simulink model "VFSIMPLEINVERTER"  (R2022b)
settings: Solver=ode1  StartTime=0.0  StopTime=10.0  FixedStep=1e-4  RelTol=1e-3
values from neighbouring files (symbols this model uses):
  f = 6.32*10.^-4    (= 0.000632)    [VFparam.m]
  J = 4.50*10.^-2    (= 0.045)    [VFparam.m]
  Kim = J*((wnm).^2)/Kpm    [VFparam.m]
  Kpm = 2*wnm*J*ceff-f    (= 2.249368)    [VFparam.m]
  Ktm = 1.5692    [VFparam.m]
  Lr = 0.2395    [VFparam.m]
  Ls = 0.256    [VFparam.m]
  Msr = 0.236    [VFparam.m]
  P = 2    [VFparam.m]
  Rr = 1.09    [VFparam.m]
  Rs = 3.36    [VFparam.m]
  VDC = 1000    [VFparam.m]
  vf = 230*sqrt(2)/50    [VFparam.m]
settings Model: Creator=ZinouAb  LastModifiedBy=ZinouAb

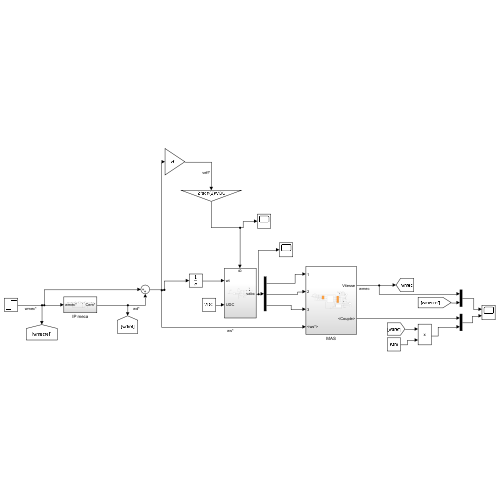
[thumbnail: Simulink's stored preview of the top-level diagram]
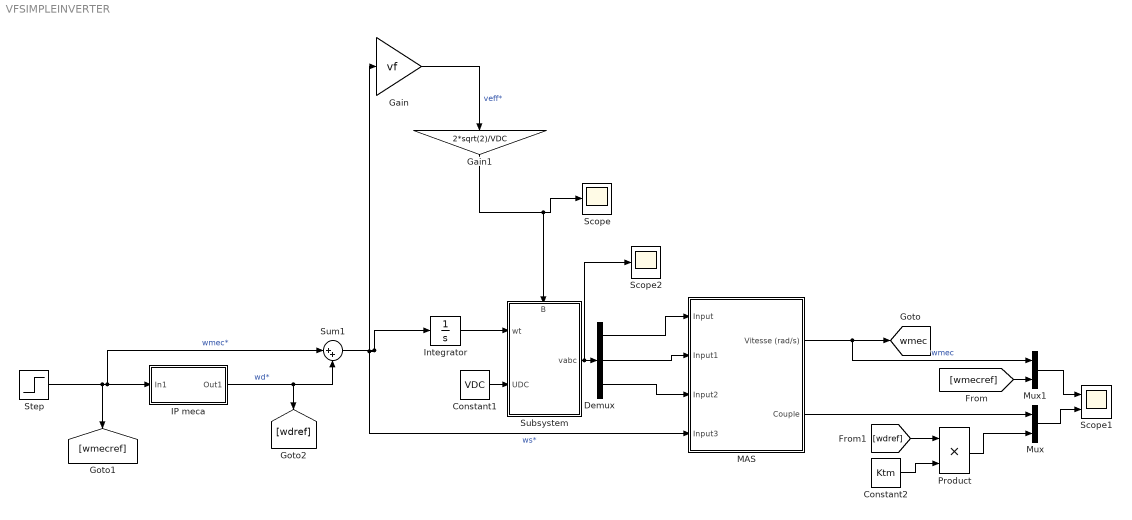
== system VFSIMPLEINVERTER ==
  Constant1 : Constant  Value=VDC
  Constant2 : Constant  Value=Ktm
  Demux : Demux  Outputs=3
  Gain : Gain  Gain=vf
  Gain1 : Gain  Gain=2*sqrt(2)/VDC
  IP meca : Subsystem
  Integrator : Integrator
  MAS : Subsystem
  Mux : Mux  Inputs=2
  Mux1 : Mux  Inputs=2
  Product : Product
  Scope : Scope
  Scope1 : Scope  NumInputPorts=2
  Scope2 : Scope
  Step : Step  Time=4  After=100  SampleTime=0
  Subsystem : Subsystem
      settings: PortSchema="{\"entries\":[{\"content\":{\"sides\":[{\"content\":{\"connectorIds\":[\"In1\",\"In2\"]},\"type\":\"ConnectorPlacement.EquallySpacedRectSide\",\"uuid\":\"b96697a1-7390-4a4c-a090-1d4840f94579\"},{\"content\":{\"connectorIds\":[\"Out1\"],\"side\":\"RIGHT\"},\"type\":\"ConnectorPlacement.EquallySpacedRectSide\",\"uuid\":\"06d1d8c6-d481-421b-9786-6ed8bea33fb5\"},{\"content\":{\"connectorIds\":[\"In3\"],\"side\":\"TOP\"},\"type\":\"ConnectorPlacement.EquallySpacedRectSide\",\"uuid\":\"2e081ee8-1238-4450-99c4-3d0e60d3e391\"}]},\"type\":\"ConnectorPlacement.EquallySpacedConnector\",\"uuid\":\"e9990dc2-fc0c-4c65-980c-f90091d8c920\"}],\"packageUris\":[\"http://schema.mathworks.com/mf0/Connector/R2020b\"],\"version\":\"1.0\"}"
  Sum1 : Sum  Inputs=|++
  tag scope: wmec=global
  wires:
  Step/1 -> IP meca/1(In1), Sum1/1, [wmecref]  "wmec*"
  Gain/1 -> Gain1/1  "veff*"
  Demux/1 -> MAS/1(Input)
  Sum1/1 -> Integrator/1, MAS/4(Input3), Gain/1  "ws*"
  Demux/2 -> MAS/2(Input1)
  MAS/1(Vitesse (rad/s)) -> Mux1/1, [wmec]  "wmec"
  Demux/3 -> MAS/3(Input2)
  IP meca/1(Out1) -> Sum1/2, [wdref]  "wd*"
  Integrator/1 -> Subsystem/1(wt)
  Subsystem/1(vabc) -> Scope2/1, Demux/1
  Constant1/1 -> Subsystem/2(UDC)
  Mux1/1 -> Scope1/1
  Mux/1 -> Scope1/2
  MAS/2(Couple) -> Mux/1
  [wmecref] -> Mux1/2
  [wdref] -> Product/1
  Constant2/1 -> Product/2
  Product/1 -> Mux/2
  Gain1/1 -> Subsystem/3(B), Scope/1

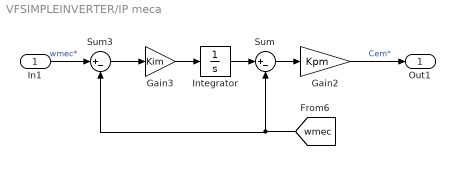
== system VFSIMPLEINVERTER/IP meca ==
  In1 : Inport
  Gain2 : Gain  Gain=Kpm
  Gain3 : Gain  Gain=Kim
  Integrator : Integrator
  Sum : Sum  Inputs=|+-
  Sum3 : Sum  Inputs=|+-
  Out1 : Outport
  wires:
  Integrator/1 -> Sum/1
  [wmec] -> Sum3/2, Sum/2
  Sum/1 -> Gain2/1
  Gain2/1 -> Out1/1  "Cem*"
  Gain3/1 -> Integrator/1
  Sum3/1 -> Gain3/1
  In1/1 -> Sum3/1  "wmec*"

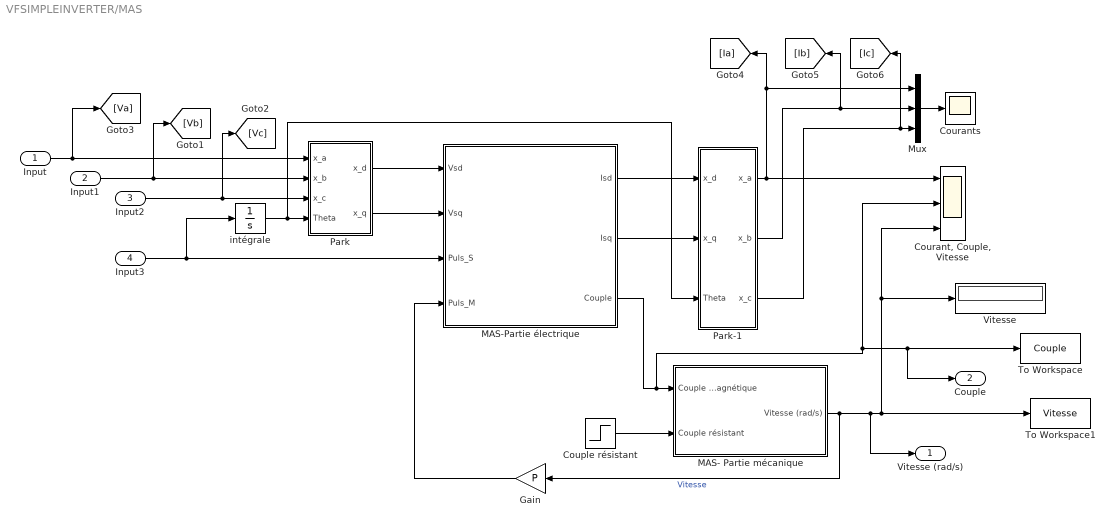
== system VFSIMPLEINVERTER/MAS ==
  Input : Inport
  Input1 : Inport  Port=2
  Input2 : Inport  Port=3
  Input3 : Inport  Port=4
  Couple résistant : Step  Time=6  After=2  SampleTime=0
  "Courant, Couple, Vitesse" : Scope  NumInputPorts=3
  Courants : Scope
  Gain : Gain  Gain=P
  MAS- Partie mécanique : Subsystem
  MAS-Partie électrique : Subsystem
  Mux : Mux  Inputs=3
  Park : Subsystem
  Park-1 : Subsystem
  To Workspace : ToWorkspace  VariableName=Couple  SampleTime=-1
      settings: Save2DSignal=2-D array (concatenate along first dimension)
  To Workspace1 : ToWorkspace  VariableName=Vitesse  SampleTime=-1
      settings: Save2DSignal=2-D array (concatenate along first dimension)
  Vitesse : Display
  intégrale : Integrator
  Vitesse (rad/s) : Outport
  Couple : Outport  Port=2
  wires:
  Park-1/2(x_b) -> [Ib], Mux/2
  Park/2(x_q) -> MAS-Partie électrique/2(Vsq)
  Input2/1 -> [Vc], Park/3(x_c)
  Mux/1 -> Courants/1
  Park-1/1(x_a) -> [Ia], Mux/1, "Courant, Couple, Vitesse"/1
  MAS- Partie mécanique/1(Vitesse (rad/s)) -> Gain/1, Vitesse (rad/s)/1, Vitesse/1, "Courant, Couple, Vitesse"/3, To Workspace1/1  "Vitesse"
  Input/1 -> [Va], Park/1(x_a)
  intégrale/1 -> Park-1/3(Theta), Park/4(Theta)
  MAS-Partie électrique/3(Couple) -> "Courant, Couple, Vitesse"/2, Couple/1, To Workspace/1, MAS- Partie mécanique/1(Couple Electromagnétique)
  Couple résistant/1 -> MAS- Partie mécanique/2(Couple résistant)
  Input1/1 -> [Vb], Park/2(x_b)
  Gain/1 -> MAS-Partie électrique/4(Puls_M)
  Park-1/3(x_c) -> [Ic], Mux/3
  Park/1(x_d) -> MAS-Partie électrique/1(Vsd)
  Input3/1 -> intégrale/1, MAS-Partie électrique/3(Puls_S)
  MAS-Partie électrique/1(Isd) -> Park-1/1(x_d)
  MAS-Partie électrique/2(Isq) -> Park-1/2(x_q)

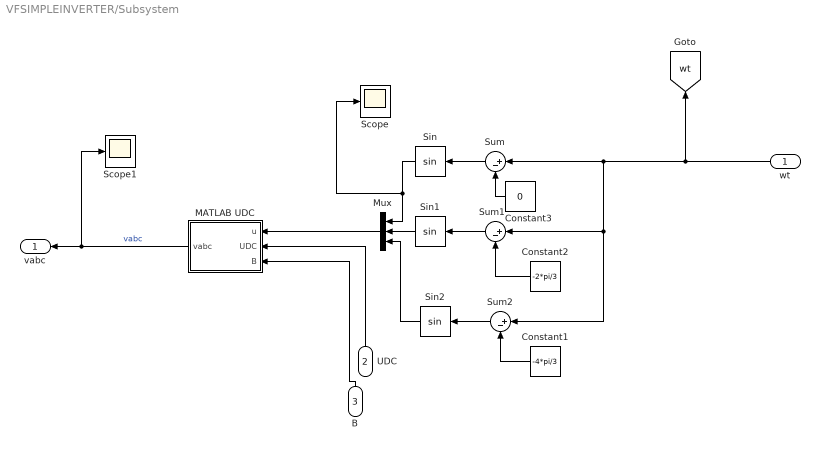
== system VFSIMPLEINVERTER/Subsystem ==
  wt : Inport
  UDC : Inport  Port=2
  B : Inport  Port=3
  Constant1 : Constant  Value=-4*pi/3
  Constant2 : Constant  Value=-2*pi/3
  Constant3 : Constant  Value=0
  MATLAB UDC : MATLAB Function  TreatAsAtomicUnit=on
  Mux : Mux  Inputs=3
  Scope : Scope
  Scope1 : Scope
  Sin : Trigonometry
  Sin1 : Trigonometry
  Sin2 : Trigonometry
  Sum : Sum  Inputs=|+-
  Sum1 : Sum  Inputs=|+-
  Sum2 : Sum  Inputs=|+-
  vabc : Outport
  tag scope: wt=global
  wires:
  Mux/1 -> MATLAB UDC/1(u)
  Sum2/1 -> Sin2/1
  Sum1/1 -> Sin1/1
  Sin1/1 -> Mux/2
  wt/1 -> [wt], Sum1/1, Sum2/1, Sum/1
  Constant2/1 -> Sum1/2
  Sin/1 -> Scope/1, Mux/1
  Sum/1 -> Sin/1
  Sin2/1 -> Mux/3
  Constant1/1 -> Sum2/2
  Constant3/1 -> Sum/2
  MATLAB UDC/1(vabc) -> Scope1/1, vabc/1  "vabc"
  B/1 -> MATLAB UDC/3(B)
  UDC/1 -> MATLAB UDC/2(UDC)

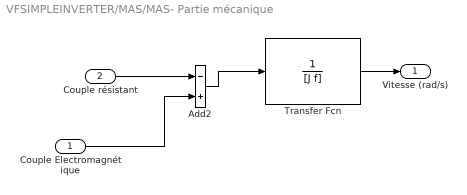
== system VFSIMPLEINVERTER/MAS/MAS- Partie mécanique ==
  Couple Electromagnétique : Inport
  Couple résistant : Inport  Port=2
  Add2 : Sum  Inputs=-+
  Transfer Fcn : TransferFcn  Denominator=[J f]
  Vitesse (rad/s) : Outport
  wires:
  Couple Electromagnétique/1 -> Add2/2
  Couple résistant/1 -> Add2/1
  Add2/1 -> Transfer Fcn/1
  Transfer Fcn/1 -> Vitesse (rad/s)/1

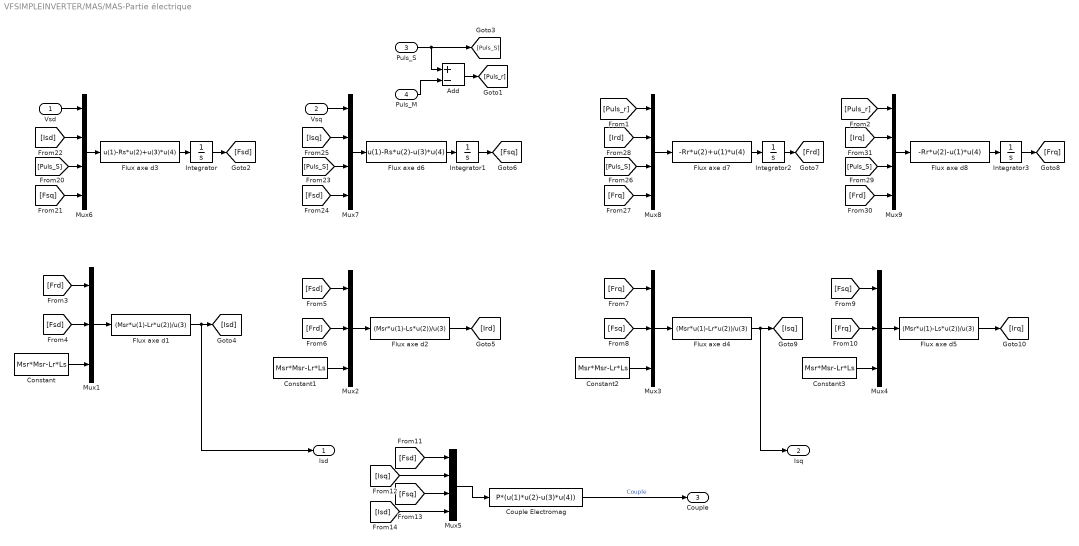
== system VFSIMPLEINVERTER/MAS/MAS-Partie électrique ==
  Vsd : Inport
  Vsq : Inport  Port=2
  Puls_S : Inport  Port=3
  Puls_M : Inport  Port=4
  Add : Sum  Inputs=+-
  Constant{,1..3} (4 alike) : Constant  Value=Msr*Msr-Lr*Ls
  Couple Electromag : Fcn  Expr=P*(u(1)*u(2)-u(3)*u(4))
  Flux axe d1 : Fcn  Expr=(Msr*u(1)-Lr*u(2))/u(3)
  Flux axe d2 : Fcn  Expr=(Msr*u(1)-Ls*u(2))/u(3)
  Flux axe d3 : Fcn  Expr=u(1)-Rs*u(2)+u(3)*u(4)
  Flux axe d4 : Fcn  Expr=(Msr*u(1)-Lr*u(2))/u(3)
  Flux axe d5 : Fcn  Expr=(Msr*u(1)-Ls*u(2))/u(3)
  Flux axe d6 : Fcn  Expr=u(1)-Rs*u(2)-u(3)*u(4)
  Flux axe d7 : Fcn  Expr=-Rr*u(2)+u(1)*u(4)
  Flux axe d8 : Fcn  Expr=-Rr*u(2)-u(1)*u(4)
  Integrator{,1..3} (4 alike) : Integrator
  Mux{1..4} (4 alike) : Mux  Inputs=3
  Mux{5..9} (5 alike) : Mux
  Isd : Outport
  Isq : Outport  Port=2
  Couple : Outport  Port=3
  wires:
  Puls_S/1 -> Add/1, [Puls_S]
  Mux6/1 -> Flux axe d3/1
  Vsd/1 -> Mux6/1
  [Isd] -> Mux6/2
  [Puls_S] -> Mux6/3
  [Fsq] -> Mux6/4
  Flux axe d3/1 -> Integrator/1
  Integrator/1 -> [Fsd]
  Mux7/1 -> Flux axe d6/1
  Vsq/1 -> Mux7/1
  [Isq] -> Mux7/2
  [Puls_S] -> Mux7/3
  [Fsd] -> Mux7/4
  Flux axe d6/1 -> Integrator1/1
  Integrator1/1 -> [Fsq]
  Mux8/1 -> Flux axe d7/1
  [Ird] -> Mux8/2
  [Puls_S] -> Mux8/3
  [Frq] -> Mux8/4
  Flux axe d7/1 -> Integrator2/1
  Integrator2/1 -> [Frd]
  Mux9/1 -> Flux axe d8/1
  [Puls_r] -> Mux8/1
  [Irq] -> Mux9/2
  [Puls_S] -> Mux9/3
  [Frd] -> Mux9/4
  Flux axe d8/1 -> Integrator3/1
  Integrator3/1 -> [Frq]
  [Puls_r] -> Mux9/1
  [Frd] -> Mux1/1
  [Fsd] -> Mux1/2
  Mux1/1 -> Flux axe d1/1
  Constant/1 -> Mux1/3
  Flux axe d1/1 -> Isd/1, [Isd]
  [Fsd] -> Mux2/1
  [Frd] -> Mux2/2
  Mux2/1 -> Flux axe d2/1
  Constant1/1 -> Mux2/3
  Flux axe d2/1 -> [Ird]
  [Frq] -> Mux3/1
  [Fsq] -> Mux3/2
  Mux3/1 -> Flux axe d4/1
  Constant2/1 -> Mux3/3
  Flux axe d4/1 -> Isq/1, [Isq]
  [Fsq] -> Mux4/1
  [Frq] -> Mux4/2
  Mux4/1 -> Flux axe d5/1
  Constant3/1 -> Mux4/3
  Flux axe d5/1 -> [Irq]
  Mux5/1 -> Couple Electromag/1
  Couple Electromag/1 -> Couple/1  "Couple"
  [Isd] -> Mux5/4
  [Fsd] -> Mux5/1
  [Isq] -> Mux5/2
  [Fsq] -> Mux5/3
  Puls_M/1 -> Add/2
  Add/1 -> [Puls_r]

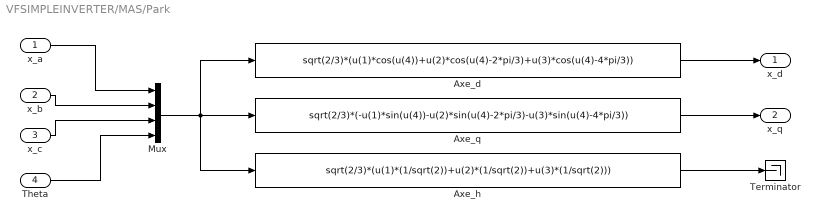
== system VFSIMPLEINVERTER/MAS/Park ==
  x_a : Inport
  x_b : Inport  Port=2
  x_c : Inport  Port=3
  Theta : Inport  Port=4
  " Axe_h" : Fcn  Expr=sqrt(2/3)*(u(1)*(1/sqrt(2))+u(2)*(1/sqrt(2))+u(3)*(1/sqrt(2)))
  " Axe_q" : Fcn  Expr=sqrt(2/3)*(-u(1)*sin(u(4))-u(2)*sin(u(4)-2*pi/3)-u(3)*sin(u(4)-4*pi/3))
  Axe_d : Fcn  Expr=sqrt(2/3)*(u(1)*cos(u(4))+u(2)*cos(u(4)-2*pi/3)+u(3)*cos(u(4)-4*pi/3))
  Mux : Mux
  Terminator : Terminator
  x_d : Outport
  x_q : Outport  Port=2
  wires:
  x_a/1 -> Mux/1
  x_b/1 -> Mux/2
  x_c/1 -> Mux/3
  Theta/1 -> Mux/4
  Mux/1 -> " Axe_q"/1, " Axe_h"/1, Axe_d/1
  " Axe_h"/1 -> Terminator/1
  " Axe_q"/1 -> x_q/1
  Axe_d/1 -> x_d/1

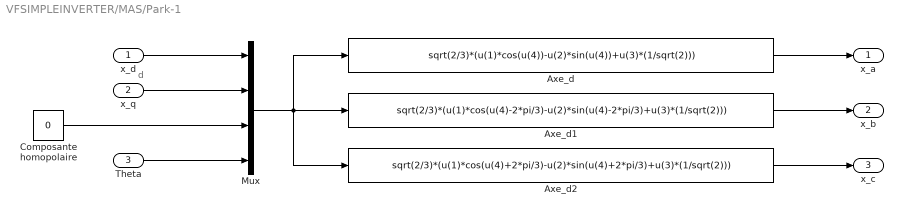
== system VFSIMPLEINVERTER/MAS/Park-1 ==
  note: d
  x_d : Inport
  x_q : Inport  Port=2
  Theta : Inport  Port=3
  Axe_d : Fcn  Expr=sqrt(2/3)*(u(1)*cos(u(4))-u(2)*sin(u(4))+u(3)*(1/sqrt(2)))
  Axe_d1 : Fcn  Expr=sqrt(2/3)*(u(1)*cos(u(4)-2*pi/3)-u(2)*sin(u(4)-2*pi/3)+u(3)*(1/sqrt(2)))
  Axe_d2 : Fcn  Expr=sqrt(2/3)*(u(1)*cos(u(4)+2*pi/3)-u(2)*sin(u(4)+2*pi/3)+u(3)*(1/sqrt(2)))
  Composante homopolaire : Constant  Value=0
  Mux : Mux
  x_a : Outport
  x_b : Outport  Port=2
  x_c : Outport  Port=3
  wires:
  x_d/1 -> Mux/1
  x_q/1 -> Mux/2
  Mux/1 -> Axe_d1/1, Axe_d2/1, Axe_d/1
  Axe_d2/1 -> x_c/1
  Axe_d1/1 -> x_b/1
  Axe_d/1 -> x_a/1
  Theta/1 -> Mux/4
  Composante homopolaire/1 -> Mux/3

== matlab function VFSIMPLEINVERTER/Subsystem/MATLAB UDC ==
  data: u input; UDC input; vabc output; B input
function vabc = gain(u,UDC,B)


vabc =0.5*UDC*B*u;
